simulink model "PWM"  (R2020b)
settings: Solver=FixedStepAuto  StartTime=0.0  StopTime=10.0  FixedStep=0.1  RelTol=1e-3
libraries: simulink x1
settings Model: Creator=petir  LastModifiedBy=petir

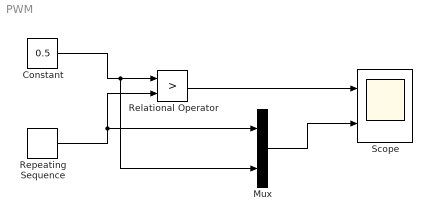
== system PWM ==
  Constant : Constant  Value=0.5
  Mux : Mux  Inputs=2
  Relational Operator : RelationalOperator  Operator=>  OutDataTypeStr=boolean  RndMeth=Simplest
  Repeating Sequence : simulink/Sources/Repeating Sequence  rep_seq_t=[0 1]  rep_seq_y=[0 1.2]
  Scope : Scope  NumInputPorts=2
  wires:
  Constant/1 -> Mux/2, Relational Operator/1
  Repeating Sequence/1 -> Relational Operator/2, Mux/1
  Mux/1 -> Scope/2
  Relational Operator/1 -> Scope/1
